simulink model "motorA"  (R2019b)
settings: Solver=VariableStepAuto  StartTime=0.0  StopTime=10.0  RelTol=1e-3
settings Model: Creator=20242496  LastModifiedBy=20242496

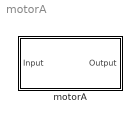
== system motorA ==
  motorA : Subsystem

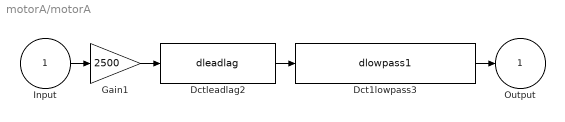
== system motorA/motorA ==
  Input : Inport
  Dct1lowpass3 : S-Function  FunctionName=dlowpass1  Parameters=f_den, 0.001  SFunctionDeploymentMode=off  EnableBusSupport=off  mask(dctools){f_den=50}
      mask prompts: f_den "Pole [Hz]"
      mask help: This block implements a discrete time 1st order lowpass filter.
      mask Display: disp('DCT 1st order lowpass')
  Dctleadlag2 : S-Function  FunctionName=dleadlag  Parameters=f_num, f_den, 0.001  SFunctionDeploymentMode=off  EnableBusSupport=off  mask(dctools){f_num=10, f_den=40}
      mask prompts: f_num "Zero [Hz]"; f_den "Pole [Hz]"
      mask help: This block implements a discrete time leadlag filter.
      mask Display: disp('DCT leadlag')
  Gain1 : Gain  Gain=2500  SaturateOnIntegerOverflow=on  OutDataTypeStr=Inherit: Same as input  ParamDataTypeStr=Inherit: Same as input
  Output : Outport
  wires:
  Input/1 -> Gain1/1
  Gain1/1 -> Dctleadlag2/1
  Dctleadlag2/1 -> Dct1lowpass3/1
  Dct1lowpass3/1 -> Output/1
